simulink model "microgrid_y24f_step3"  (R2024b)
settings: Solver=ode45  StartTime=0.0  StopTime=simu.endTime  MaxStep=simu.maxStepSize  RelTol=1e-3
undefined symbols (not defined in the file or in its folder): wt
settings Model: Creator=tedbrekken  LastModifiedBy=kerrychen
settings RTWCC: GPUComputeCapability=3.5

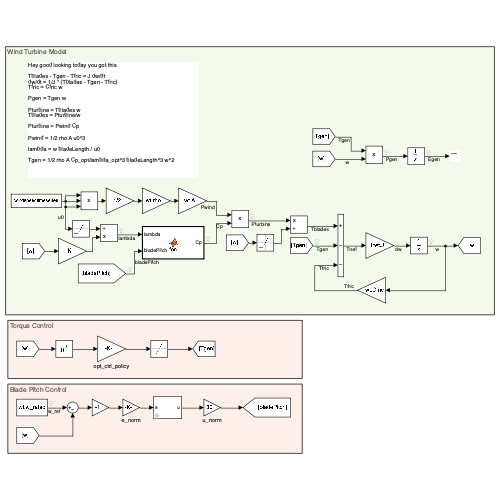
[thumbnail: Simulink's stored preview of the top-level diagram]
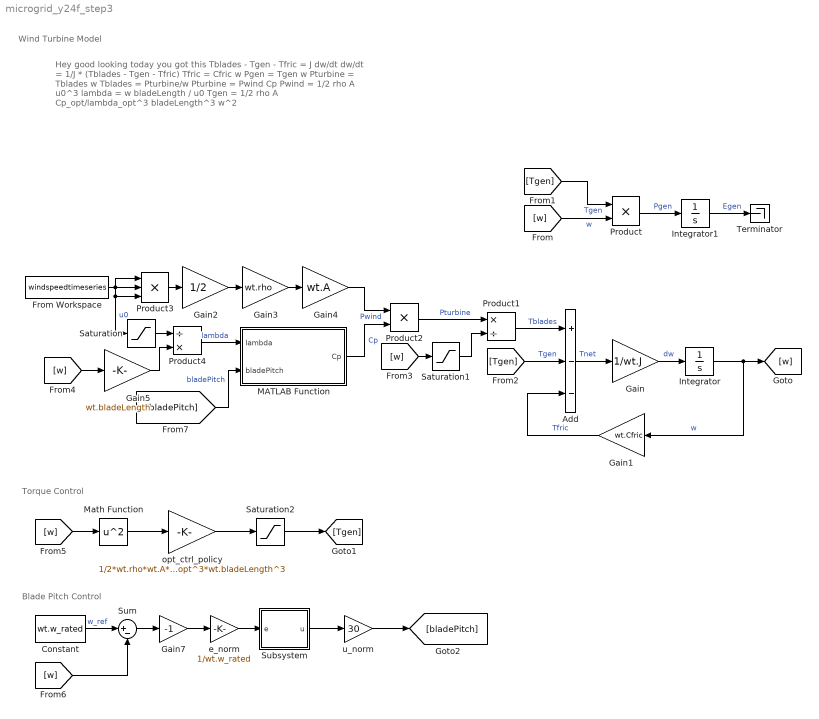
== system microgrid_y24f_step3 ==
  note: Blade Pitch Control
  note: Wind Turbine Model
  note: Hey good looking today you got this
      |
      | Tblades - Tgen - Tfric = J dw/dt
      | dw/dt = 1/J * (Tblades - Tgen - Tfric)
      | Tfric = Cfric w
      |
      | Pgen = Tgen w
      |
      | Pturbine = Tblades w
      | Tblades = Pturbine/w
      |
      | Pturbine = Pwind Cp
      |
      | Pwind = 1/2 rho A u0^3
      |
      | lambda = w bladeLength / u0
      |
      | Tgen = 1/2 rho A Cp_opt/lambda_opt^3 bladeLength^3 w^2
  note: Torque Control
  Add : Sum  Inputs=+--
  Constant : Constant  Value=wt.w_rated
  From Workspace : FromWorkspace  VariableName=windspeedtimeseries
  Gain : Gain  Gain=1/wt.J
  Gain1 : Gain  Gain=wt.Cfric
  Gain2 : Gain  Gain=1/2
  Gain3 : Gain  Gain=wt.rho
  Gain4 : Gain  Gain=wt.A
  Gain5 : Gain  Gain=wt.bladeLength
  Gain7 : Gain  Gain=-1
  Integrator : Integrator  InitialCondition=wt.w_0
  Integrator1 : Integrator
  MATLAB Function : MATLAB Function  TreatAsAtomicUnit=on
  Math Function : Math  Operator=square
  Product : Product
  Product1 : Product  Inputs=*/
  Product2 : Product
  Product3 : Product  Inputs=3
  Product4 : Product  Inputs=/*
  Saturation : Saturate  UpperLimit=inf  LowerLimit=1e-3
  Saturation1 : Saturate  UpperLimit=inf  LowerLimit=1e-3
  Saturation2 : Saturate  UpperLimit=wt.Tgen_rated  LowerLimit=0
  Subsystem : Subsystem  mask{kp=wt.pitchctrl.kp, ki=wt.pitchctrl.ki, upperLimit=wt.pitchctrl.upperLimit, lowerLimit=wt.pitchctrl.lowerLimit}
      mask prompts: kp "Proportional gain"; ki "Integral gain"; upperLimit "Upper limit"; lowerLimit "Lower limit"
  Sum : Sum  Inputs=|+-
  Terminator : Terminator
  e_norm : Gain  Gain=1/wt.w_rated
  opt_ctrl_policy : Gain  Gain=1/2*wt.rho*wt.A*wt.Cp_opt/wt.lambda_opt^3*wt.bladeLength^3
  u_norm : Gain  Gain=30
  wires:
  Product1/1 -> Add/1  "Tblades"
  [Tgen] -> Add/2  "Tgen"
  Add/1 -> Gain/1  "Tnet"
  Gain/1 -> Integrator/1  "dw"
  Integrator/1 -> [w], Gain1/1  "w"
  Gain1/1 -> Add/3  "Tfric"
  [Tgen] -> Product/1  "Tgen"
  [w] -> Product/2  "w"
  Product/1 -> Integrator1/1  "Pgen"
  Product2/1 -> Product1/1  "Pturbine"
  MATLAB Function/1(Cp) -> Product2/2  "Cp"
  Gain2/1 -> Gain3/1
  Gain3/1 -> Gain4/1
  Gain4/1 -> Product2/1  "Pwind"
  Product3/1 -> Gain2/1
  Gain5/1 -> Product4/2
  [w] -> Gain5/1
  From Workspace/1 -> Saturation/1, Product3/3, Product3/2, Product3/1  "u0"
  Product4/1 -> MATLAB Function/1(lambda)  "lambda"
  Saturation/1 -> Product4/1
  [w] -> Saturation1/1
  Saturation1/1 -> Product1/2
  [w] -> Math Function/1
  [bladePitch] -> MATLAB Function/2(bladePitch)  "bladePitch"
  opt_ctrl_policy/1 -> Saturation2/1
  Math Function/1 -> opt_ctrl_policy/1
  Saturation2/1 -> [Tgen]
  Constant/1 -> Sum/1  "w_ref"
  [w] -> Sum/2
  Subsystem/1(u) -> u_norm/1
  Sum/1 -> Gain7/1
  Gain7/1 -> e_norm/1
  e_norm/1 -> Subsystem/1(e)
  u_norm/1 -> [bladePitch]
  Integrator1/1 -> Terminator/1  "Egen"

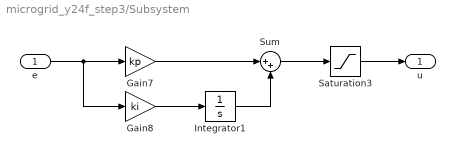
== system microgrid_y24f_step3/Subsystem ==
  e : Inport
  Gain7 : Gain  Gain=kp
  Gain8 : Gain  Gain=ki
  Integrator1 : Integrator  LimitOutput=on  UpperSaturationLimit=upperLimit  LowerSaturationLimit=lowerLimit
  Saturation3 : Saturate  UpperLimit=upperLimit  LowerLimit=lowerLimit
  Sum : Sum  Inputs=|++
  u : Outport
  wires:
  Integrator1/1 -> Sum/2
  Saturation3/1 -> u/1
  e/1 -> Gain8/1, Gain7/1
  Gain8/1 -> Integrator1/1
  Gain7/1 -> Sum/1
  Sum/1 -> Saturation3/1

== matlab function microgrid_y24f_step3/MATLAB Function ==
  data: lambda input; Cp output; bladePitch input
function Cp = fcn(lambda,bladePitch)

% https://www.mathworks.com/help/physmod/sps/powersys/ref/windturbine.html

c = [...
    0.5176 ...
    116 ...
    0.4 ...
    5 ...
    21 ...
    0.0068];

if (lambda+0.08*bladePitch) == 0
    lambda = 1e-3;
end

lambdaai = 1/( 1/(lambda+0.08*bladePitch) - 0.035/(bladePitch^3+1) );

Cp = c(1)*(c(2)/lambdaai-c(3)*bladePitch-c(4))*exp(-c(5)/lambdaai) + c(6)*lambda;
